simulink model "LKAS"  (R2018b)
settings: Solver=FixedStepDiscrete  StartTime=0.0  StopTime=10.0  FixedStep=0.01  RelTol=1e-3
InitFcn:
  | tmpVer = ver('MATLAB');
  | tmpVer = str2num(tmpVer.Version);
  | % -------------------------------------------------------------------
  | %  MATLAB file generated by Simulink.saveVars on 21-Nov-2019 10:06:14
  | %  MATLAB version: 7.13.0.564 (R2011b)
  | % -------------------------------------------------------------------
  | 
  | 
  | SInt16 = Simulink.AliasType;
  | SInt16.Description = 'Num';
  | if (tmpVer > 7.11)
  | 	SInt16.DataScope = 'Auto';
  | end
  | SInt16.HeaderFile = 'Rte_Type.h';
  | SInt16.BaseType = 'int16';
  | 
  | SInt32 = Simulink.AliasType;
  | SInt32.Description = 'Num';
  | if (tmpVer > 7.11)
  | 	SInt32.DataScope = 'Auto';
  | end
  | SInt32.HeaderFile = 'Rte_Type.h';
  | SInt32.BaseType = 'int32';
  | 
  | SInt8 = Simulink.AliasType;
  | SInt8.Description = 'Num';
  | if (tmpVer > 7.11)
  | 	SInt8.DataScope = 'Auto';
  | end
  | SInt8.HeaderFile = 'Rte_Type.h';
  | SInt8.BaseType = 'int8';
  | 
  | T_A_m2_1024_1_u32 = Simulink.NumericType;
  | T_A_m2_1024_1_u32.Description = 'm2 (square meters  (m2))';
  | if (tmpVer > 7.11)
  | 	T_A_m2_1024_1_u32.DataScope = 'Auto';
  | end
  | T_A_m2_1024_1_u32.HeaderFile = 'Rte_Type.h';
  | T_A_m2_1024_1_u32.DataTypeMode = 'Fixed-point: slope and bias scaling';
  | T_A_m2_1024_1_u32.SignednessBool = false;
  | T_A_m2_1024_1_u32.WordLength = 32;
  | T_A_m2_1024_1_u32.FixedExponent = -10;
  | T_A_m2_1024_1_u32.SlopeAdjustmentFactor = 1;
  | T_A_m2_1024_1_u32.Bias = 0;
  | T_A_m2_1024_1_u32.DataTypeOverride = 'Inherit';
  | T_A_m2_1024_1_u32.IsAlias = true;
  | 
  | T_A_m2_65536_1_u16 = Simulink.NumericType;
  | T_A_m2_65536_1_u16.Description = 'm2 (square meters  (m2))';
  | if (tmpVer > 7.11)
  | 	T_A_m2_65536_1_u16.DataScope = 'Auto';
  | end
  | T_A_m2_65536_1_u16.HeaderFile = 'Rte_Type.h';
  | T_A_m2_65536_1_u16.DataTypeMode = 'Fixed-point: slope and bias scaling';
  | T_A_m2_65536_1_u16.SignednessBool = false;
  | T_A_m2_65536_1_u16.WordLength = 16;
  | T_A_m2_65536_1_u16.FixedExponent = -16;
  | T_A_m2_65536_1_u16.SlopeAdjustmentFactor = 1;
  | T_A_m2_65536_1_u16.Bias = 0;
  | T_A_m2_65536_1_u16.DataTypeOverride = 'Inherit';
  | ... (+4598 lines)
StopFcn:
  | clear  T_A_m2_1024_1_u32 T_A_m2_65536_1_u16 T_A_m2_Float32 T_A_mm2_10_1_u16 T_A_mm2_4_1_s16 T_A_mm2_Float32 T_Cnt_Num_10_1_u32 T_Cnt_Num_1_1_s16 T_Cnt_Num_1_1_s32 T_Cnt_Num_1_1_s8 T_Cnt_Num_1_1_u16 T_Cnt_Num_1_1_u32 T_Cnt_Num_1_1_u8 T_E_J_1_1_s32 T_E_J_Float32 T_E_kJ_128_1_s32 T_E_kJ_Float32 T_E_kwh_10_1_u16 T_E_kwh_Float32 T_Epl_kwhpkm_100_1_u16 T_Epl_kwhpkm_Float32 T_F_N_1_1_s16 T_F_N_Float32 T_I_A_1000_1_u16 T_I_A_1048576_1_s32 T_I_A_2048_1_s16 T_I_A_32_1_s16 T_I_A_Float32 T_I_mA_1_1_s16 T_I_mA_32768_128_s16 T_I_mA_Float32 T_J_kgpm2_128_1_u16 T_J_kgpm2_Float32 T_K_NA_1000_1_s16 T_K_NA_100_1_s16 T_K_NA_100_1_u16 T_K_NA_1024_1_s16 T_K_NA_1024_1_u16 T_K_NA_128_1_s16 T_K_NA_128_1_u16 T_K_NA_128_1_u8 T_K_NA_16777216_1_u32 T_K_NA_16_1_s16 T_K_NA_16_1_u16 T_K_NA_16_1_u8 T_K_NA_1_16_u16 T_K_NA_1_1_s16 T_K_NA_1_1_u16 T_K_NA_1_1_u8 T_K_NA_32768_1_s16 T_K_NA_32768_1_u16 T_K_NA_32_1_s8 T_K_NA_4096_1_u16 T_K_NA_4194304_1_s32 T_K_NA_4194304_1_u16 T_K_NA_65536_1_s32 T_K_NA_65536_1_u16 T_K_NA_8192_1_s16 T_K_NA_8_1_s16 T_K_NA_Float32 T_M_Nm_16_1_s16 T_M_Nm_1_1_s16 T_M_Nm_32768_1_s16 T_M_Nm_32_1_s16 T_M_Nm_4_1_s16 T_M_Nm_512_1_s16 T_M_Nm_Float32 T_P_W_1_4_s16 T_P_W_1_8_s16 T_P_W_Float32 T_P_kW_128_1_s16 T_P_kW_1_8_s16 T_P_kW_8_1_s32 T_P_kW_Float32 T_Pct_pct_1024_1_s32 T_Pct_pct_1024_1_u32 T_Pct_pct_10_1_s16 T_Pct_pct_10_1_u32 T_Pct_pct_128_100_s8 T_Pct_pct_1_1_s16 T_Pct_pct_1_4_u8 T_Pct_pct_255_100_u16 T_Pct_pct_255_100_u8 T_Pct_pct_256_1_s16 T_Pct_pct_256_1_u16 T_Pct_pct_65535_100_u16 T_Pct_pct_Float32 T_R_ohm_1024_1_s16 T_R_ohm_32_1_s16 T_R_ohm_Float32 T_TK_K_16_1_s16 T_TK_K_Float32 T_T_degC_10_400_1_u16 T_T_degC_16_1_s16 T_T_degC_1_40_1_u8 T_T_degC_2_80_1_u8 T_T_degC_Float32 T_U_V_1000_1_u16 T_U_V_10_1_u8 T_U_V_200_1_u8 T_U_V_32_1_s16 T_U_V_4096_1_s16 T_U_V_512_1_s16 T_U_V_65535_8_u16 T_U_V_8192_1_u16 T_U_V_Float32 T_U_mV_1_1_s16 T_U_mV_256_20_u16 T_U_mV_Float32 T_V_l_256_1_s16 T_V_l_4096_1_s16 T_V_l_64_1_s16 T_V_l_65535_100_u16 T_V_l_Float32 T_V_ml_128_1_s16 T_V_ml_1_1_s16 T_V_ml_32768_1_s16 T_V_ml_Float32 T_V_ul_32_1_u16 T_V_ul_Float32 T_Vpl_clpkm_512_1_u16 T_Vpl_clpkm_Float32 T_a_kphps_16_1_s16 T_a_kphps_Float32 T_a_mps2_128_1_s16 T_a_mps2_Float32 T_c_MJpkg_256_1_s16 T_c_MJpkg_Float32 T_c_kJpgpK_1024_1_s16 T_c_kJpgpK_Float32 T_c_kJpkgpK_128_1_u16 T_c_kJpkgpK_Float32 T_chrg_Ah_1_1_s16 T_chrg_Ah_1_1_u16 T_chrg_Ah_1_1_u8 T_chrg_Ah_256_1_u16 T_chrg_Ah_4194304_1_s32 T_chrg_Ah_512_1_u16 T_chrg_Ah_8_1_u16 T_chrg_Ah_Float32 T_cmp_NA_100_1_s16 T_cmp_NA_128_1_s16 T_cmp_NA_16_1_s16 T_cmp_NA_32768_1_u16 T_cmp_NA_Float32 T_d2n_rpmps2_4_1_s16 T_d2n_rpmps2_Float32 T_dPct_pctps_16_1_s16 T_dPct_pctps_256_1_s16 T_dPct_pctps_Float32 T_dT_degCps_128_1_s16 T_dT_degCps_Float32 T_dV_lph_1_1_s16 T_dV_lph_Float32 T_dV_lpm_128_1_s16 T_dV_lpm_32_1_s16 T_dV_lpm_Float32 T_dV_lps_1024_1_u16 T_dV_lps_4_1_u16 T_dV_lps_Float32 T_dV_mlps_1024_1_s16 T_dV_mlps_Float32 T_d_BitField16 T_dm_gps_128_1_s16 T_dm_gps_128_1_u16 T_dm_gps_256_1_u16 T_dm_gps_Float32 T_dm_mgps_1_1_s16 T_dm_mgps_Float32 T_dn_rpmps_1_1_s16 T_dn_rpmps_2_1_s16 T_dn_rpmps_Float32 T_dp_Paps_1_1_s16 T_dp_Paps_Float32 T_dp_kPaps_1_1_s16 T_dp_kPaps_8_1_s16 T_dp_kPaps_Float32 T_dphi_degps_128_1_s16 T_dphi_degps_8_1_s16 T_dphi_degps_Float32 T_dr_ps_256_1_s16 T_dr_ps_Float32 T_drho_mgplps_1_2_s16 T_drho_mgplps_Float32 T_e_NA_1_1_u8 T_f_Hz_1_1_u16 T_f_Hz_1_1_u32 T_f_Hz_64_1_u16 T_f_Hz_8_1_s16 T_f_Hz_Float32 T_g_BitField32 T_l_km_16_1_s16 T_l_km_1_1_u16 T_l_km_1_1_u32 T_l_km_Float32 T_l_m_1024_1_s16 T_l_m_16_1_s16 T_l_m_1_1_u32 T_l_m_Float32 T_l_mm_16_1_s16 T_l_mm_1_1_u16 T_l_mm_4096_1_s16 T_l_mm_4_1_u8 T_l_mm_64_1_s16 T_l_mm_Float32 T_m_g_1_1_s16 T_m_g_2048_1_s16 T_m_g_32_1_u16 T_m_g_Float32 T_m_kg_1024_1_s16 T_m_kg_1_1_s16 T_m_kg_1_1_u32 T_m_kg_Float32 T_m_mg_128_1_s16 T_m_mg_32_1_s16 T_m_mg_Float32 T_n_rpm_1_1_s16 T_n_rpm_1_25_u8 T_n_rpm_256_50_u16 T_n_rpm_2_25_u8 T_n_rpm_4_1_u16 T_n_rpm_Float32 T_p_MPa_64_1_s16 T_p_MPa_Float32 T_p_Pa_1_1_s16 T_p_Pa_Float32 T_p_kPa_1_10_u16 T_p_kPa_1_1_s16 T_p_kPa_1_1_u8 T_p_kPa_256_1_u16 T_p_kPa_32_1_u16 T_p_kPa_64_1_s16 T_p_kPa_Float32 T_phi_deg_100_1_s16 T_phi_deg_1024_1_s16 T_phi_deg_128_1_s16 T_phi_deg_1_1_u8 T_phi_deg_256_1_s16 T_phi_deg_2_1_s8 T_phi_deg_32_1_s16 T_phi_deg_512_6_s32 T_phi_deg_Float32 T_phi_rad_2048_1_s16 T_phi_rad_Float32 T_r_NA_1024_1_s16 T_r_NA_1024_1_u16 T_r_NA_16384_1_s16 T_r_NA_16_1_s16 T_r_NA_256_1_s8 T_r_NA_256_1_u16 T_r_NA_32768_1_u16 T_r_NA_32_1_u16 T_r_NA_4096_1_s16 T_r_NA_65535_2_u16 T_r_NA_8192_1_u16 T_r_NA_Float32 T_rho_gpl_8192_1_s16 T_rho_gpl_Float32 T_rho_kgpm3_16_1_s16 T_rho_kgpm3_Float32 T_rho_mgpl_1_1_s16 T_rho_mgpl_64_1_s16 T_rho_mgpl_Float32 T_t_hour_1_1_s16 T_t_hour_Float32 T_t_m_1_1_u16 T_t_m_Float32 T_t_ms_1_1_s16 T_t_ms_1_1_u16 T_t_ms_1_1_u32 T_t_ms_4096_1_s16 T_t_ms_64_1_s16 T_t_ms_Float32 T_t_s_1000_1_s16 T_t_s_100_1_s16 T_t_s_10_1_s16 T_t_s_10_1_u16 T_t_s_1_1_s16 T_t_s_1_1_u16 T_t_s_1_1_u32 T_t_s_Float32 T_t_us_10_1_u32 T_t_us_1_1_s16 T_t_us_1_1_u32 T_t_us_1_4_u16 T_t_us_Float32 T_v_kph_1_1_u8 T_v_kph_64_1_s16 T_v_kph_64_1_u16 T_v_kph_Float32 T_v_mps_256_1_s16 T_v_mps_Float32 T_w_radps_32_1_s16 T_w_radps_Float32 T_y_BitField8 T_y_BitFieldDiagProgress T_y_BitFieldDiagStatus T_y_NA_1_1_u8 SInt16 SInt32 SInt8 T_BOOLEAN UInt16 UInt32 UInt8 s16 s32 s8 u16 u32 u8
model workspace (MAT data in the model file):
  MCOS : class17 (value not decoded)
  MCOS : class17 (value not decoded)
  MCOS : class17 (value not decoded)
  MCOS : class17 (value not decoded)
  MCOS : class17 (value not decoded)
  MCOS : class17 (value not decoded)
  MCOS : class17 (value not decoded)
  MCOS : class17 (value not decoded)
  MCOS : class17 (value not decoded)
  MCOS : class17 (value not decoded)
  MCOS : class17 (value not decoded)
  MCOS : class17 (value not decoded)
  MCOS : class17 (value not decoded)
  MCOS : class17 (value not decoded)
  MCOS : class17 (value not decoded)
  MCOS : class17 (value not decoded)
  MCOS : class17 (value not decoded)
  MCOS : class17 (value not decoded)
  MCOS : class17 (value not decoded)
  MCOS : class17 (value not decoded)
  MCOS : class17 (value not decoded)
  MCOS : class17 (value not decoded)
  MCOS : class17 (value not decoded)
  MCOS : class17 (value not decoded)
  MCOS : class17 (value not decoded)
  MCOS : class17 (value not decoded)
  MCOS : class17 (value not decoded)
  MCOS : class17 (value not decoded)
  MCOS : class17 (value not decoded)
  MCOS : class17 (value not decoded)
  MCOS : class17 (value not decoded)
  MCOS : class17 (value not decoded)
  MCOS : class17 (value not decoded)
  MCOS : class17 (value not decoded)
  MCOS : class17 (value not decoded)
  MCOS : class17 (value not decoded)
  MCOS : class17 (value not decoded)
  MCOS : class17 (value not decoded)
  MCOS : class17 (value not decoded)
  MCOS : class17 (value not decoded)
  MCOS : class17 (value not decoded)
  MCOS : class17 (value not decoded)
  MCOS : class17 (value not decoded)
  MCOS : class17 (value not decoded)
  MCOS : class17 (value not decoded)
  MCOS : class17 (value not decoded)
  MCOS : class17 (value not decoded)
  MCOS : class17 (value not decoded)
  MCOS : class17 (value not decoded)
  MCOS : class17 (value not decoded)
  MCOS : class17 (value not decoded)
  MCOS : class17 (value not decoded)
  MCOS : class17 (value not decoded)
  MCOS : class17 (value not decoded)
  MCOS : class17 (value not decoded)
  MCOS : class17 (value not decoded)
  MCOS : class17 (value not decoded)
  MCOS : class17 (value not decoded)
  MCOS : class17 (value not decoded)
  MCOS : class17 (value not decoded)
  MCOS : class17 (value not decoded)
  MCOS : class17 (value not decoded)
  MCOS : class17 (value not decoded)
  MCOS : class17 (value not decoded)
  MCOS : class17 (value not decoded)
  MCOS : class17 (value not decoded)
  MCOS : class17 (value not decoded)
  MCOS : class17 (value not decoded)
  MCOS : class17 (value not decoded)
  MCOS : class17 (value not decoded)
  MCOS : class17 (value not decoded)
  MCOS : class17 (value not decoded)
  MCOS : class17 (value not decoded)
  MCOS : class17 (value not decoded)
  MCOS : class17 (value not decoded)
  MCOS : class17 (value not decoded)
  MCOS : class17 (value not decoded)
  MCOS : class17 (value not decoded)
  MCOS : class17 (value not decoded)
  MCOS : class17 (value not decoded)
  MCOS : class17 (value not decoded)
  MCOS : class17 (value not decoded)
  MCOS : class17 (value not decoded)
  MCOS : class17 (value not decoded)
  MCOS : class17 (value not decoded)
  MCOS : class17 (value not decoded)
  MCOS : class17 (value not decoded)
  MCOS : class17 (value not decoded)
  MCOS : class17 (value not decoded)
undefined symbols (not defined in the file): LKA_CarWidth, LKA_SampleTime, LKA_StrRatio_C, LKA_Veh2CamL_C, LKA_Veh2CamW_C, LKA_WhlBaseL_C, LL_CompSWA_C, LL_CrvtPrvwT_C, LL_DesDvt_C, LL_DvtComp_C, LL_DvtPrvwT_C, LL_DvtSpdDet_vDvtSpdMin_C, LL_HdAgExT_C, LL_HdAgPrvwT_C, LL_LAccMax_C, LL_LAccRMax_C, LL_LDW_EarliestWarnLine_C, LL_LDW_LatestWarnLine_C, LL_LDWS_SUPPRESS_HEADING, LL_LFClb_TFC_DiffCtlBalance, LL_LFClb_TFC_DiffCtrlMaxSWA, LL_LFClb_TFC_DiffCtrlRatio, LL_LFClb_TFC_facmGainLutGain1_C, LL_LFClb_TFC_facmGainLutGain2_C, LL_LFClb_TFC_facmIntegRatio, LL_LFClb_TFC_facmKlat_C, LL_LFClb_TFC_FfCtlRatio_C, LL_LFClb_TFC_phiIntegCtlMaxSWA_C, LL_LFClb_TFC_tiKlatPrvwT_C, LL_LFClb_TFC_vGainLutVehSpdLwr_C, LL_LFClb_TFC_vGainLutVehSpdUpr_C, LL_LKA_EarliestWarnLine_C, LL_LKA_LatestWarnLine_C, LL_LKAExPrcs_ExitC0Dvt, LL_LKAExPrcs_ExitC0Swt, LL_LKAExPrcs_tiExitTime1, LL_LKAExPrcs_tiExitTime2, LL_LKAExPrcs_tiExitTime3, LL_LKAS_OUT_OF_CONTROL_LAT_VEL, LL_LKAS_OUT_OF_CONTROL_TTLC, LL_LKASWASyn_M0, LL_LKASWASyn_M1, LL_LKASWASyn_M2, LL_LKASWASyn_M3K, LL_LKASWASyn_SWAaddMax, LL_LKASWASyn_T2, LL_LKASWASyn_tiTrqSwaRtTime, LL_LKASWASyn_tiTrqSwaTime, LL_LKASWASyn_TrqMax, LL_LKASWASyn_TrqSwaAddSwt, LL_LKASWASyn_TrqSwaRateDiff, LL_LSpdCompT_C, LL_lStpLngth_C, LL_MAX_DELAY_EPSSTAR_TIME, LL_MAX_DRIVER_TORQUE_DISABLE, LL_MAX_DRIVER_TORQUE_ENABLE, LL_MAX_LANE_WIDTH_DISABLE, LL_MAX_LANE_WIDTH_ENABLE, LL_MAX_LAT_ACC_DISABLE, LL_MAX_LAT_ACC_ENABLE ... (+29)
libraries: simulink x190, dspstat3 x3, simulink_extras x1
(part 7 of 19)

== system LKAS/LKAS/LL/LL Inputs Mapping/bsLaneInfo/LanesReconstruct  ==
  bsL0Info : Inport
  bsR0Info : Inport  Port=2
  bsL1Info : Inport  Port=3
  bsR1Info : Inport  Port=4
  Bus Selector5 : BusSelector  OutputSignals=L0_Q
  Bus Selector6 : BusSelector  OutputSignals=R0_Q
  LaneReconstructSM : Stateflow chart  TreatAsAtomicUnit=on
  Left 1Lane Reconstruct (Lft1LaneR) : Subsystem
  Left Lane Reconstruct (LftLaneR) : Subsystem
  Right 1Lane Reconstruct (Rgt1LaneR) : Subsystem
  Right Lane Reconstruct (RgtLaneR) : Subsystem
  RoadSide Offset : Subsystem
  Switch : Switch  Criteria=u2 > Threshold
  Switch1 : Switch  Criteria=u2 > Threshold
  bsL0InfoR : Outport
  bsR0InfoR : Outport  Port=2
  bsL1InfoR : Outport  Port=3
  bsR1InfoR : Outport  Port=4
  wires:
  RoadSide Offset/2(bsR0Infoout) -> Bus Selector6/1, Left Lane Reconstruct (LftLaneR)/2(bsR0Info), Right Lane Reconstruct (RgtLaneR)/2(bsR0Info), Switch/1
  RoadSide Offset/1(bsL0Infoout) -> Bus Selector5/1, Right Lane Reconstruct (RgtLaneR)/1(bsL0Info), Switch1/1, Left Lane Reconstruct (LftLaneR)/3(bsL0Info)
  bsL0Info/1 -> RoadSide Offset/1(bsL0Info)
  bsR0Info/1 -> RoadSide Offset/2(bsR0Info)
  [LftFlg] -> Switch1/2
  [RgtFlg] -> Switch/2
  [LftFlg] -> Left 1Lane Reconstruct (Lft1LaneR)/1(stFlag)
  [RgtFlg] -> Right 1Lane Reconstruct (Rgt1LaneR)/1(stFlag)
  Left 1Lane Reconstruct (Lft1LaneR)/1(bsL1InfoR) -> bsL1InfoR/1
  Right 1Lane Reconstruct (Rgt1LaneR)/1(bsL1InfoR) -> bsR1InfoR/1
  bsR1Info/1 -> Right 1Lane Reconstruct (Rgt1LaneR)/2(bsR1Info)
  LaneReconstructSM/3(LaneRSM_stRgtFlg) -> [RgtFlg]
  LaneReconstructSM/2(LaneRSM_stLftFlg) -> [LftFlg]
  LaneReconstructSM/1(LaneRSM_stRoadFlg) -> [RoadFlg]
  Switch1/1 -> bsL0InfoR/1
  Switch/1 -> bsR0InfoR/1
  Right Lane Reconstruct (RgtLaneR)/1(bsR0InfoR) -> Switch/3
  Left Lane Reconstruct (LftLaneR)/1(bsL0InfoR) -> Switch1/3
  RoadSide Offset/3(lRoadW) -> Right Lane Reconstruct (RgtLaneR)/3(lRoadW), Left Lane Reconstruct (LftLaneR)/1(lRoadW), [RoadWidth]
  Bus Selector5/1 -> LaneReconstructSM/1(LaneRSM_stL0Ql)  "<L0_Q>"
  Bus Selector6/1 -> LaneReconstructSM/2(LaneRSM_stR0Ql)  "<R0_Q>"
  bsL1Info/1 -> Left 1Lane Reconstruct (Lft1LaneR)/2(bsL1Info)

== system LKAS/LKAS/LL/LLOn/LDW/Heading Angle Detection (HdAgDet) ==
  HdAgDet_stLDWActvFlg : Inport
  HdAgDet_phiHdAgLft : Inport  Port=2
  HdAgDet_phiHdAgRgt : Inport  Port=3
  HdAgDet_phiHdAgThres_C : Inport  Port=4
  Constant : Constant  Value=5  OutDataTypeStr=single
  If : If  IfExpression=u1==1  ElseIfExpressions=u1==2
  If Action Subsystem : Subsystem  TreatAsAtomicUnit=on
  If Action Subsystem1 : Subsystem  TreatAsAtomicUnit=on
  If Action Subsystem2 : Subsystem  TreatAsAtomicUnit=on
  Merge : Merge  Inputs=3  InitialOutput=0
  Relational Operator : RelationalOperator  OutDataTypeStr=boolean  RndMeth=Nearest
  Sum Condition : Subsystem
  HdAgDet_stHdAgDetFlg : Outport
  wires:
  If/1 -> If Action Subsystem/Action
  If Action Subsystem/1(Out1) -> Merge/1
  If Action Subsystem1/1(Out1) -> Merge/2
  If/2 -> If Action Subsystem1/Action
  If Action Subsystem2/1(Out1) -> Merge/3
  If/3 -> If Action Subsystem2/Action
  HdAgDet_phiHdAgLft/1 -> If Action Subsystem/1(In1)
  HdAgDet_phiHdAgRgt/1 -> If Action Subsystem1/1(In1)
  HdAgDet_stLDWActvFlg/1 -> If/1
  Merge/1 -> Relational Operator/1
  HdAgDet_phiHdAgThres_C/1 -> Relational Operator/2
  Sum Condition/1(Out) -> HdAgDet_stHdAgDetFlg/1
  Relational Operator/1 -> Sum Condition/1(In), Sum Condition/Enable
  Constant/1 -> Sum Condition/2(Sum)

== system LKAS/LKAS/LL/LLOn/LKA/Driver Torque Addition (DTA) ==
  DTA_bsInInfoSyn : Inport
  DTA_bsLFClb : Inport  Port=2
  Bus Selector : BusSelector  OutputSignals=LL_LKASWAClb.LL_LKASWASyn_TrqSwaAddSwt
  Compare To Constant : simulink/Logic and Bit Operations/Compare To Constant  relop=>  const=0  OutDataTypeStr=boolean
  Subsystem : Subsystem
  Subsystem1 : Subsystem
  DTA_phiDTASWACmd : Outport
  DTA_M : Outport  Port=2
  wires:
  [LKA_SampleTime] -> Subsystem/3(LKA_SampleTime)
  DTA_bsInInfoSyn/1 -> Subsystem/1(DTA_bsInInfoSyn), Subsystem1/1(DTA_bsInInfoSyn)
  DTA_bsLFClb/1 -> Subsystem1/2(DTA_bsLFClb), Subsystem/2(DTA_bsLFClb), Bus Selector/1
  Subsystem/1(Out1) -> DTA_phiDTASWACmd/1
  Subsystem1/1(Out1) -> DTA_M/1
  Bus Selector/1 -> Compare To Constant/1  "<LL_LKASWASyn_TrqSwaAddSwt>"
  Compare To Constant/1 -> Subsystem/Enable

== system LKAS/LKAS/LL/LLOn/LKA/LKA Exit Processing (LKAExPrcs) ==
  LKAExPrcs_bsInInfoSyn : Inport
  LKAExPrcs_bsLKAInPInfo : Inport  Port=2
  LKAExPrcs_bsLKAClb : Inport  Port=3
  LKAExPrcs_PlanT1 : Inport  Port=4
  Cast To Single : DataTypeConversion  OutDataTypeStr=single
  Exit Time 1 : Subsystem
  Exit Time 2 : Subsystem
  Exit Time 3 : Subsystem
  Fcn : Fcn  Expr=u(3)*(u(3)==1)*3+u(2)*(u(3)==0)*2+u(1)*(u(2)==0&&u(3)==0)
  Logical Operator3 : Logic  Operator=OR  Inputs=3  AllPortsSameDT=off  OutDataTypeStr=boolean
  Mux : Mux  Inputs=3
  LKAExPrcs_stExFlg : Outport
  LKAExPrcs_stExNum : Outport  Port=2
  wires:
  LKAExPrcs_bsInInfoSyn/1 -> Exit Time 3/1(bsInInfoSyn), Exit Time 2/1(bsInInfoSyn)
  Logical Operator3/1 -> LKAExPrcs_stExFlg/1
  Exit Time 1/1(Exit1) -> Mux/1, Logical Operator3/1
  Exit Time 2/1(Exit2) -> Mux/2, Logical Operator3/2
  Exit Time 3/1(Exit3) -> Mux/3, Logical Operator3/3
  LKAExPrcs_bsLKAInPInfo/1 -> Exit Time 3/2(bsLKAInPInfo), Exit Time 2/3(bsLKAInPInfo), Exit Time 1/1(bsLKAInPInfo)
  LKAExPrcs_bsLKAClb/1 -> Exit Time 1/2(bsLKAClb), Exit Time 2/2(bsLKAClb), Exit Time 3/3(bsLKAClb)
  LKAExPrcs_PlanT1/1 -> Exit Time 2/4(T1), Exit Time 3/4(T1)
  Mux/1 -> Cast To Single/1
  Fcn/1 -> LKAExPrcs_stExNum/1  "ExNum"
  Cast To Single/1 -> Fcn/1

== system LKAS/LKAS/LL/LLOn/LKA/LKA Motion Planning (LKAMP)  ==
  LKAMP_bsInInfoSyn : Inport
  LKAMP_stLKAActvFlg : Inport  Port=2
  LKAMP_bsLKAInPInfo : Inport  Port=3
  LKAMP_bsLKAClb : Inport  Port=4
  LLClb_bsConstantClb : Inport  Port=5
  Add : Sum  OutDataTypeStr=uint8
  Bus Selector : BusSelector  OutputSignals=MPInP_vVehSpdIni
  Bus Selector1 : BusSelector  OutputSignals=bsVehMovInfo.ESC_VehSpd
  Bus Selector2 : BusSelector  OutputSignals=LKA_CarWidth
  Bus Selector3 : BusSelector  OutputSignals=LL_HdAgExT_C,LL_LSpdCompT_C
  Bus Selector4 : BusSelector  OutputSignals=bsVehMovInfo.ESC_VehSpd
  Bus Selector5 : BusSelector  OutputSignals=LW_LaneWidth
  Constant : Constant  OutDataTypeStr=uint8  SampleTime=-1
  Constant19 : Constant  OutDataTypeStr=uint8  SampleTime=-1
  If : If  NumInputs=2  IfExpression=u1==u2  ShowElse=off
  LKA Motion Planning Calculation (LKAMPCal) : Subsystem  Description=|
      | Block Name: LKA Motion Planning Calculation
      | Ab.: LKAMPCal
      | No.: 1.2.3.2
      | Rev: 0.0.1
      | Update Date: 19-3-26
      settings: RTWSystemCode=Nonreusable function
  Memory1 : Memory  InheritSampleTime=on
  Motion Planning Input Processing (MPInP) : Subsystem  Description=|
      | Block Name: Motion Planning Input Processing
      | Ab.: MPInP
      | No.: 1.2.3.1
      | Rev: 0.0.1
      | Update Date: 19-3-26
  Nominal Time Calculation (NomTCalc) : Subsystem  Description=|
      | Block Name: Nominal Time Calculation
      | Ab.: NomTCalc
      | No.: 1.2.3.3
      | Rev: 0.0.1
      | Update Date: 19-3-26
  Saturation1 : Saturate  UpperLimit=5  LowerLimit=0  OutDataTypeStr=uint8
  Saturation6 : Saturate  UpperLimit=2  LowerLimit=0.2
  Steering Wheel Angle Command Calculation (SWACmdCal) : Subsystem  Description=|
      | Block Name: Steering Wheel Angle Command Calculation
      | Ab.: SWACmdCal
      | No.: 1.2.3.4
      | Rev: 0.0.1
      | Update Date: 19-3-26
  Switching Condition (SwtCon) : Subsystem
  LKAMP_phiSWACmd : Outport
  LKAMP_tiT1 : Outport  Port=2
  LKAMP_tiT2 : Outport  Port=3
  wires:
  Steering Wheel Angle Command Calculation (SWACmdCal)/3(SWACmdCal_tiT2) -> LKAMP_tiT2/1
  Motion Planning Input Processing (MPInP)/1(MPInP_bsMPInPInfo) -> Steering Wheel Angle Command Calculation (SWACmdCal)/2(SWACmdCal_bsLKAInPInfo), Bus Selector/1, LKA Motion Planning Calculation (LKAMPCal)/1(LKAMPCal_bsLKAInPInfo)  "LKAMP_bsMPInPInfo"
  Steering Wheel Angle Command Calculation (SWACmdCal)/2(SWACmdCal_tiT1) -> Saturation6/1
  Steering Wheel Angle Command Calculation (SWACmdCal)/1(SWACmdCal_phiSWACmd) -> LKAMP_phiSWACmd/1
  Bus Selector/1 -> Nominal Time Calculation (NomTCalc)/2(NomTCalc_vVehSpdIni)  "<MPInP_vVehSpdIni>"
  Bus Selector1/1 -> Nominal Time Calculation (NomTCalc)/1(NomTCalc_vVehSpd)  "<ESC_VehSpd>"
  Nominal Time Calculation (NomTCalc)/1(NomTCalc_tiNomT) -> Steering Wheel Angle Command Calculation (SWACmdCal)/3(SWACmdCal_tiNomT)
  Switching Condition (SwtCon)/1(SwtCon_phiHdAgMax) -> Motion Planning Input Processing (MPInP)/2(MPInP_phiHdAgMax)
  LKA Motion Planning Calculation (LKAMPCal)/1(LKAMPCal_bsLKAMPCalOut) -> Steering Wheel Angle Command Calculation (SWACmdCal)/1(SWACmdCal_bsK1K2DetOut)
  If/1 -> LKA Motion Planning Calculation (LKAMPCal)/Action
  Memory1/1 -> Add/2
  Constant/1 -> Add/1
  Constant19/1 -> If/2
  Add/1 -> Saturation1/1
  Saturation1/1 -> Memory1/1, If/1
  Bus Selector3/1 -> Switching Condition (SwtCon)/6(SwtCon_tiHdAgExTime_C)  "<LL_HdAgExT_C>"
  Bus Selector4/1 -> Switching Condition (SwtCon)/3(SwtCon_vVehSpd)  "<ESC_VehSpd>"
  LKAMP_stLKAActvFlg/1 -> Switching Condition (SwtCon)/1(SwtCon_stLKAActvFlg), Motion Planning Input Processing (MPInP)/1(MPInP_stLKAActvFlg)
  LKAMP_bsLKAClb/1 -> Bus Selector3/1, LKA Motion Planning Calculation (LKAMPCal)/2(LKAMPCal_bsLKAClb)
  Bus Selector2/1 -> Switching Condition (SwtCon)/5(SwtCon_lCarWidth_C)  "<LKA_CarWidth>"
  LKAMP_bsLKAInPInfo/1 -> Bus Selector5/1, Switching Condition (SwtCon)/2(SwtCon_bsLKAInPInfo), Motion Planning Input Processing (MPInP)/3(MPInP_bsLKAInPInfo)
  LLClb_bsConstantClb/1 -> LKA Motion Planning Calculation (LKAMPCal)/3(LLClb_bsConstantClb), Bus Selector2/1
  Bus Selector3/2 -> Switching Condition (SwtCon)/7(SwtCon_tiLSpdCompT_C)  "<LL_LSpdCompT_C>"
  LKAMP_bsInInfoSyn/1 -> Motion Planning Input Processing (MPInP)/4(MPInP_bsInInfoSyn), Bus Selector1/1, Bus Selector4/1
  Saturation6/1 -> LKAMP_tiT1/1
  Bus Selector5/1 -> Switching Condition (SwtCon)/4(SwtCon_lLaneWidth_C)  "<LW_LaneWidth>"

== system LKAS/LKAS/LL/LLOn/LKA/LKA SWA Limit (LKASWALim) ==
  LKASWALim_phiTFCSWACmd : Inport
  LKASWALim_Ff : Inport  Port=2
  LKASWALim_bsLKAInPInfo : Inport  Port=3
  LKASWALim_bsLKAClb : Inport  Port=4
  Add : Sum  Inputs=+-+  OutDataTypeStr=single
  Add1 : Sum
  Add2 : Sum
  Bus Selector1 : BusSelector  OutputSignals=LKAInP_phiSWAPos,UndrLim_phiSWAMax,UndrLim_dphiSWARMax
  Bus Selector3 : BusSelector  OutputSignals=LL_CompSWA_C
  Gain1 : Gain  Gain=-1.4  OutDataTypeStr=single
  Gain2 : Gain  Gain=-1  OutDataTypeStr=single
  Gain3 : Gain  Gain=1.4  OutDataTypeStr=single
  "Rate Limiter Dynamic " : Subsystem
  Saturation Dynamic : simulink/Discontinuities/Saturation Dynamic  OutMin=[]  OutMax=[]  OutDataTypeStr=Inherit: Same as second input  OutDataType=fixdt(1, 16)  OutScaling=2^-10  DoSatur=off
  LKASWALim_phiSWACmd : Outport
  wires:
  Gain3/1 -> "Rate Limiter Dynamic "/1(up)
  Saturation Dynamic/1 -> "Rate Limiter Dynamic "/2(u)
  "Rate Limiter Dynamic "/1(Y) -> LKASWALim_phiSWACmd/1
  Bus Selector3/1 -> Add/2  "<LL_CompSWA_C>"
  LKASWALim_phiTFCSWACmd/1 -> Add/1
  LKASWALim_bsLKAClb/1 -> Bus Selector3/1
  Bus Selector1/2 -> Add1/2, Gain2/1  "<UndrLim_phiSWAMax>"
  Bus Selector1/3 -> Gain3/1, Gain1/1  "<UndrLim_dphiSWARMax>"
  Gain2/1 -> Add2/2
  Gain1/1 -> "Rate Limiter Dynamic "/3(lo)
  Add/1 -> Saturation Dynamic/2
  LKASWALim_bsLKAInPInfo/1 -> Bus Selector1/1
  Bus Selector1/1 -> Add/3  "<LKAInP_phiSWAPos>"
  LKASWALim_Ff/1 -> Add2/1, Add1/1
  Add1/1 -> Saturation Dynamic/1
  Add2/1 -> Saturation Dynamic/3

== system LKAS/LKAS/LL/LLOn/LKA/Lane Following (LF) ==
  LF_bsInInfoSyn : Inport
  LF_bsLKAInPInfo : Inport  Port=2
  LF_bsLFClb : Inport  Port=3
  LF_bsConstantClb : Inport  Port=4
  Bus Selector4 : BusSelector  OutputSignals=LL_TFCClb
  Preview Information Calculation (PIC) : Subsystem  Description=|
      | Block Name:Preview Information Calculation
      | Ab.: PIC
      | No.: 02.01
      | Rev: 00.00.01
      | Update Date: 19-3-28
  Trajectory Following Control (TFC) : Subsystem  Description=|
      | Block Name:Trajectory Following Control
      | Ab.: TFC
      | No.: 02.02
      | Rev: 00.00.01
      | Update Date: 19-3-28
  LF_phiFfLFSWACmd : Outport
  LF_phiPropSWACmd : Outport  Port=2
  LF_phiIntegSWACmd : Outport  Port=3
  LF_phiDiffSWACmd : Outport  Port=4
  wires:
  Trajectory Following Control (TFC)/4(TFC_phiDiffSWACmd) -> LF_phiDiffSWACmd/1
  Trajectory Following Control (TFC)/3(TFC_phiIntegSWACmd) -> LF_phiIntegSWACmd/1
  Trajectory Following Control (TFC)/2(TFC_phiPropSWACmd) -> LF_phiPropSWACmd/1
  LF_bsConstantClb/1 -> Trajectory Following Control (TFC)/4(TFC_bsConstantClb)
  LF_bsLFClb/1 -> Bus Selector4/1
  Bus Selector4/1 -> Trajectory Following Control (TFC)/3(TFC_bsTFCClb)  "<LL_TFCClb>"
  Preview Information Calculation (PIC)/1(PIC_bsPrvwInfo) -> Trajectory Following Control (TFC)/1(TFC_bsPrvwInfo)
  LF_bsInInfoSyn/1 -> Trajectory Following Control (TFC)/2(TFC_bsInInfoSyn)
  Trajectory Following Control (TFC)/1(TFC_phiFfSWACmd) -> LF_phiFfLFSWACmd/1
  LF_bsLKAInPInfo/1 -> Preview Information Calculation (PIC)/1(PIC_bsLKAInPInfo)

== system LKAS/LKAS/LL/LLOn/LKA/Plan To LaneFollowing (PTLF) ==
  InP : Inport
  Plan : Inport  Port=2
  T1 : Inport  Port=3
  DrvTrq : Inport  Port=4
  Ff : Inport  Port=5
  P : Inport  Port=6
  I : Inport  Port=7
  D : Inport  Port=8
  Add1 : Sum  Inputs=+-
  Add2 : Sum  Inputs=+-
  Add3 : Sum
  Add4 : Sum  Inputs=+++++
  Add5 : Sum  Inputs=+-
  Bus Selector1 : BusSelector  OutputSignals=Pr_bsPrInfo.bsPrCrvtInfo.crPrvwCrvt
  Bus Selector2 : BusSelector  OutputSignals=Pr_bsPrInfo.bsPrHdAgInfo.phiHdAgLft,Pr_bsPrInfo.bsPrHdAgInfo.phiHdAgRgt
  Constant1 : Constant  Value=0.1  OutDataTypeStr=single
  Constant2 : Constant  OutDataTypeStr=single
  Divide : Product  Inputs=*/
  Divide{1..2,5..7} (5 alike) : Product  Inputs=**
  Divide3 : Product  Inputs=*/
  Divide4 : Product  Inputs=*/
  InsideJudge : Subsystem
  InsideJudge1 : Subsystem
  LowPass : Subsystem
  Saturation : Saturate  UpperLimit=1  LowerLimit=0
  Saturation1 : Saturate  UpperLimit=1  LowerLimit=0
  Saturation2 : Saturate  UpperLimit=1  LowerLimit=0
  Saturation3 : Saturate  UpperLimit=0.004  LowerLimit=-0.004
  Saturation6 : Saturate  LowerLimit=0.2
  Switch : Switch  Criteria=u2 > Threshold
  TickTime (TTime) : Subsystem
      mask Display:
      | port_label('output', 1, 'TTime');
      | color('blue');
      | text(0.98,0.9,'VCDC Block','horizontalAlignment','right');
      | color('black');
      | text(0.5,0.55,'Tick Time','horizontalAlignment','center');
      | text(0.5,0.4,'(TTime)','horizontalAlignment','center');
  TimeGain : Subsystem
  SWACmd : Outport
  wires:
  Constant1/1 -> LowPass/1(T)
  [LKA_SampleTime] -> LowPass/3(dT)
  LowPass/1(y) -> SWACmd/1
  Divide2/1 -> Add4/3  "S_D"
  Divide4/1 -> Saturation1/1
  Divide1/1 -> Add4/2  "S_PI"
  Add3/1 -> Divide1/2
  I/1 -> Add3/2
  P/1 -> Add3/1
  Divide7/1 -> Add4/1  "S_Plan"
  DrvTrq/1 -> Divide6/1
  D/1 -> Divide2/1
  Ff/1 -> Divide5/2
  Add5/1 -> Divide7/2
  Divide6/1 -> Add4/5  "S_DT"
  [Plan] -> Divide7/1
  Saturation2/1 -> Divide1/1, Add5/2
  Constant2/1 -> Add5/1
  Saturation/1 -> Divide6/2
  Divide/1 -> Saturation2/1
  Divide3/1 -> Saturation/1
  [T1] -> Add2/2
  Add2/1 -> Divide/1
  Add4/1 -> LowPass/2(u)
  [TFC] -> Divide/2
  Saturation1/1 -> Divide2/2
  Bus Selector1/1 -> Saturation3/1  "<crPrvwCrvt>"
  Saturation3/1 -> InsideJudge/2(Crvt)
  Divide5/1 -> Switch/3, Switch/1
  TimeGain/1(Out1) -> Divide5/1
  TickTime (TTime)/1(Out1) -> [Time]
  [ActFlg] -> InsideJudge/1(Flg)
  InsideJudge/1(Out1) -> Switch/2
  Switch/1 -> Add4/4  "S_Ff"
  [Time] -> Divide3/1
  [Time] -> Add2/1
  [T1] -> Divide3/2
  InsideJudge1/1(T1_1) -> [T1], Saturation6/1
  Saturation6/1 -> [TFC]
  [Time] -> TimeGain/1(Time)
  [T1] -> TimeGain/2(T1)
  [TFC] -> TimeGain/3(TFC)
  [T1] -> Add1/2
  [TFC] -> Divide4/2
  Add1/1 -> Divide4/1
  [Time] -> Add1/1
  InP/1 -> Bus Selector2/1, Bus Selector1/1
  [ActFlg] -> InsideJudge1/1(Flg)
  Bus Selector2/1 -> InsideJudge1/2(HdAgLft)  "<phiHdAgLft>"
  Bus Selector2/2 -> InsideJudge1/3(HdAgRgt)  "<phiHdAgRgt>"
  T1/1 -> InsideJudge1/4(T1)
  Plan/1 -> InsideJudge1/5(Plan)
  [Time] -> InsideJudge1/6(Time)
  InsideJudge1/2(Plan_1) -> [Plan]

== system LKAS/LKAS/LL/LLOn/LKA Input Processing (LKAInP)/Lane Width Calculation (LW) ==
  LW_bsInInfoSyn : Inport
  Abs : Abs
  Abs1 : Abs
  Add : Sum
  Bus Selector : BusSelector  OutputSignals=bsLaneInfo.bsL0Info.L0_C0,bsLaneInfo.bsR0Info.R0_C0
  Saturation : Saturate  UpperLimit=6  LowerLimit=2
  LW_LaneWidth : Outport
  wires:
  LW_bsInInfoSyn/1 -> Bus Selector/1
  Bus Selector/1 -> Abs/1  "<L0_C0>"
  Bus Selector/2 -> Abs1/1  "<R0_C0>"
  Abs/1 -> Add/1
  Abs1/1 -> Add/2
  Add/1 -> Saturation/1
  Saturation/1 -> LW_LaneWidth/1  "LaneWidth"

== system LKAS/LKAS/LL/LLOn/LKA Input Processing (LKAInP)/Predicted Deviation Calculation (PrDvt) ==
  PrdcDvt_stLKAActvFlg : Inport
  PrdcDvt_bsInInfoSyn : Inport  Port=2
  PrdcDvt_bsPrdcHdAgInfo : Inport  Port=3
  PrdcDvt_bsLKAClb : Inport  Port=4
  Bus Creator1 : BusCreator  Inputs=8
  Bus Selector : BusSelector  OutputSignals=bsLaneInfo.bsL0Info,bsVehMovInfo.ESC_VehSpd,bsLaneInfo.bsR0Info
  Bus Selector1 : BusSelector  OutputSignals=LL_DvtPrvwT_C,LL_DvtComp_C
  Bus Selector2 : BusSelector  OutputSignals=bsLaneInfo.bsL0Info.L0_C0,bsLaneInfo.bsR0Info.R0_C0
  Bus Selector3 : BusSelector  OutputSignals=EnaCClb.LL_DvtComp_C
  Lane Information Selection (LaneInfoSel) : Subsystem
  Lane Information Selection (LaneInfoSel)1 : Subsystem
  Left Front Conner Deviation Calculation (LFCDvtCalc) : Subsystem
  Predicted Deviation Correction (PrdcDvtCor) : Subsystem
  Predicted Deviation of Left Lane Line (PrdcDvtLft) : Subsystem
  Predicted Deviation of Left Line (PrdcDvtLft) : Subsystem
  Predicted Deviation of Right  Line (PrdcDvtRgt) : Subsystem
  Predicted Deviation of Right Lane Line (PrdcDvtRgt) : Subsystem
  Right Front Conner Deviation Calculation (RFCDvtCalc) : Subsystem
  Z Calculation (ZCalc) : Subsystem
  PrdcDvt_bsPrdcDvtInfo : Outport
  wires:
  Bus Selector1/2 -> Predicted Deviation of Left Line (PrdcDvtLft)/4(PrdcDvtLft_lDvtComp_C), Predicted Deviation of Right  Line (PrdcDvtRgt)/4(PrdcDvtLft_lDvtComp_C)  "<LL_DvtComp_C>"
  Bus Selector1/1 -> Z Calculation (ZCalc)/2(ZCalc_tiDvtPrvwT_C)  "<LL_DvtPrvwT_C>"
  PrdcDvt_bsLKAClb/1 -> Bus Selector1/1
  Predicted Deviation Correction (PrdcDvtCor)/1(PrdcDvtCor_lPrdcDvtCor) -> Predicted Deviation of Right  Line (PrdcDvtRgt)/2(PrdcDvtLft_lPrdcDvtCor), Predicted Deviation of Left Line (PrdcDvtLft)/2(PrdcDvtLft_lPrdcDvtCor)
  PrdcDvt_bsPrdcHdAgInfo/1 -> Right Front Conner Deviation Calculation (RFCDvtCalc)/3(PrdcDvt_bsPrHdAgInfo), Left Front Conner Deviation Calculation (LFCDvtCalc)/1(PrdcDvt_bsPrHdAgInfo), Predicted Deviation Correction (PrdcDvtCor)/1(PrdcDvtCor_bsPrdcHdAgInfo), Predicted Deviation of Right  Line (PrdcDvtRgt)/1(PrdcDvtLft_bsPrdcHdAgInfo), Predicted Deviation of Left Line (PrdcDvtLft)/1(PrdcDvtLft_bsPrdcHdAgInfo)
  Bus Selector/1 -> Predicted Deviation of Left Lane Line (PrdcDvtLft)/1(PrdcDvtLft_bsL0Info)  "<bsL0Info>"
  PrdcDvt_bsInInfoSyn/1 -> Bus Selector2/1, Bus Selector/1
  Z Calculation (ZCalc)/1(ZCalc_lPrvwDstZ) -> Predicted Deviation of Right Lane Line (PrdcDvtRgt)/1(PrdcDvtRgt_lPrvwDstZ), Predicted Deviation of Left Lane Line (PrdcDvtLft)/2(PrdcDvtLft_lPrvwDstZ), Predicted Deviation Correction (PrdcDvtCor)/2(PrdcDvtCor_lPrvwDstZ)
  Predicted Deviation of Right Lane Line (PrdcDvtRgt)/1(PrdcDvtRgt_lPrdcDvtRgt) -> Bus Creator1/5, Predicted Deviation of Right  Line (PrdcDvtRgt)/3(PrdcDvtLft_lPrdcDvtLft)  "lPrvwDvtRgt"
  Bus Selector/2 -> Z Calculation (ZCalc)/1(ZCalc_vVehSpd)  "<ESC_VehSpd>"
  Bus Selector/3 -> Predicted Deviation of Right Lane Line (PrdcDvtRgt)/2(PrdcDvtRgt_bsR0Info)  "<bsR0Info>"
  Predicted Deviation of Left Lane Line (PrdcDvtLft)/1(PrdcDvtLft_lPrdcDvtLft) -> Bus Creator1/4, Predicted Deviation of Left Line (PrdcDvtLft)/3(PrdcDvtLft_lPrdcDvtLft)  "lPrvwDvtLft"
  Predicted Deviation of Left Line (PrdcDvtLft)/1(PrdcDvtLft_lDvtLft) -> Bus Creator1/2, Lane Information Selection (LaneInfoSel)/2(LaneInfoSel_facmLftLane)  "lPrdcDvtLft"
  Predicted Deviation of Right  Line (PrdcDvtRgt)/1(PrdcDvtLft_lDvtRgt) -> Lane Information Selection (LaneInfoSel)/3(LaneInfoSel_facmRgtLane), Bus Creator1/3  "lPrdcDvtRgt"
  Bus Creator1/1 -> PrdcDvt_bsPrdcDvtInfo/1
  PrdcDvt_stLKAActvFlg/1 -> Lane Information Selection (LaneInfoSel)/1(LaneInfoSel_stLKAActvFlg), Lane Information Selection (LaneInfoSel)1/1(LaneInfoSel_stLKAActvFlg)
  Lane Information Selection (LaneInfoSel)/1(LaneInfoSel_facmActvLane) -> Bus Creator1/1  "lPrdcDvt"
  Bus Selector2/1 -> Left Front Conner Deviation Calculation (LFCDvtCalc)/2(LFCDvtCalc_lDvt)  "<L0_C0>"
  Bus Selector2/2 -> Right Front Conner Deviation Calculation (RFCDvtCalc)/2(RFCDvtCalc_lDvt)  "<R0_C0>"
  [LLClb_bsLLSMConClb] -> Bus Selector3/1
  Bus Selector3/1 -> Right Front Conner Deviation Calculation (RFCDvtCalc)/1(RFCDvtCalc_lDvtComp_C), Left Front Conner Deviation Calculation (LFCDvtCalc)/3(LFCDvtCalc_lDvtComp_C)  "<LL_DvtComp_C>"
  Left Front Conner Deviation Calculation (LFCDvtCalc)/1(DvtCalc_lLftDvt) -> Lane Information Selection (LaneInfoSel)1/2(LaneInfoSel_facmLftLane), Bus Creator1/7  "ILftDvt"
  Right Front Conner Deviation Calculation (RFCDvtCalc)/1(DvtCalc_lRgtDvt) -> Lane Information Selection (LaneInfoSel)1/3(LaneInfoSel_facmRgtLane), Bus Creator1/8  "IRgtDvt"
  Lane Information Selection (LaneInfoSel)1/1(LaneInfoSel_facmActvLane) -> Bus Creator1/6  "lDvt"

== system LKAS/LKAS/LL/LLOn/LKA Input Processing (LKAInP)/Predicted Heading Angle Calculation (PrHdAg) ==
  PrHdAg_bsTTLCInfo : Inport
  PrdcHdAg_stLKAActvFlg : Inport  Port=2
  PrHdAg_bsInInfoSyn : Inport  Port=3
  PrHdAg_bsLKAClb : Inport  Port=4
  Add : Sum  OutDataTypeStr=single
  Add1 : Sum  OutDataTypeStr=single
  Bus Creator : BusCreator  Inputs=10
  Bus Selector : BusSelector  OutputSignals=bsLaneInfo.bsL0Info,bsVehMovInfo.ESC_VehSpd,bsLaneInfo.bsR0Info,bsSWAInfo.SW_Angle
  Bus Selector1 : BusSelector  OutputSignals=LL_HdAgPrvwT_C
  Bus Selector2 : BusSelector  OutputSignals=LFTTTLC,RGTTTLC
  Heading Angle (HdAg) : Subsystem
  Lane Information Selection (LaneInfoSel) : Subsystem
  Lane Information Selection (LaneInfoSel)1 : Subsystem
  Min : MinMax  Inputs=2
  Perdicted Heading Angle Compensation (PrdcHdAgComp) : Subsystem
  Perdicted Heading Angle from Right Lane Line (PrdcHdAgRgt) : Subsystem
  Perdicted Heading Angle from Right Lane Line (PrdcHdAgRgt)1 : Subsystem
  Predicted Heading Angle from Left Lane Line (PrdcHdAgtLft) : Subsystem
  Predicted Heading Angle from Left Lane Line (PrdcHdAgtLft)1 : Subsystem
  Saturation : Saturate  UpperLimit=2  LowerLimit=0.5
  Z Calculation (ZCalc) : Subsystem
  Z Calculation (ZCalc)1 : Subsystem
  PrHdAg_bsPrHdAgInfo : Outport
  wires:
  Min/1 -> Saturation/1
  Bus Selector/4 -> Perdicted Heading Angle Compensation (PrdcHdAgComp)/2(PrdcHdAgComp_phiSWA)  "<SW_Angle>"
  Bus Selector/3 -> Perdicted Heading Angle from Right Lane Line (PrdcHdAgRgt)1/2(PrdcHdAgRgt_bsR0Info), Perdicted Heading Angle from Right Lane Line (PrdcHdAgRgt)/2(PrdcHdAgRgt_bsR0Info)  "<bsR0Info>"
  Bus Selector/2 -> Z Calculation (ZCalc)1/1(ZCalc_vVehSpd), Perdicted Heading Angle Compensation (PrdcHdAgComp)/1(PrdcHdAgComp_vVehSpd), Z Calculation (ZCalc)/1(ZCalc_vVehSpd)  "<ESC_VehSpd>"
  PrHdAg_bsInInfoSyn/1 -> Heading Angle (HdAg)/1(HdAg_bsLaneInfo), Bus Selector/1
  Bus Creator/1 -> PrHdAg_bsPrHdAgInfo/1
  Perdicted Heading Angle from Right Lane Line (PrdcHdAgRgt)/1(PrdcHdAgRgt_phiPrdcHdAgRgt) -> Bus Creator/4, Lane Information Selection (LaneInfoSel)1/3(LaneInfoSel_facmRgtLane), Add1/1  "phiPrvwTTLCHdAgRgt"
  Predicted Heading Angle from Left Lane Line (PrdcHdAgtLft)/1(PrdcHdAgtLft_phiPrdcHdAgLft) -> Lane Information Selection (LaneInfoSel)1/2(LaneInfoSel_facmLftLane), Bus Creator/3, Add/1  "phiPrvwTTLCHdAgLft"
  Perdicted Heading Angle Compensation (PrdcHdAgComp)/1(PrdcHdAgComp_phiPrdcHdAgComp) -> Add/2, Bus Creator/5, Add1/2  "phiPrdcHdAgComp"
  Add/1 -> Lane Information Selection (LaneInfoSel)/2(LaneInfoSel_facmLftLane)  "phiPrdcHdAgLft"
  Add1/1 -> Lane Information Selection (LaneInfoSel)/3(LaneInfoSel_facmRgtLane)  "phiPrdcHdAgRgt"
  PrdcHdAg_stLKAActvFlg/1 -> Lane Information Selection (LaneInfoSel)1/1(LaneInfoSel_stLKAActvFlg), Lane Information Selection (LaneInfoSel)/1(LaneInfoSel_stLKAActvFlg)
  Lane Information Selection (LaneInfoSel)/1(LaneInfoSel_facmActvLane) -> Bus Creator/1  "phiPrdcTTLCHdAg"
  Z Calculation (ZCalc)/1(ZCalc_lPrvwDstZ) -> Perdicted Heading Angle from Right Lane Line (PrdcHdAgRgt)/1(PrdcHdAgRgt_lPrvwDstZ), Predicted Heading Angle from Left Lane Line (PrdcHdAgtLft)/2(PrdcHdAgtLft_lPrvwDstZ)
  Bus Selector/1 -> Predicted Heading Angle from Left Lane Line (PrdcHdAgtLft)1/1(PrdcHdAgtLft_bsL0Info), Predicted Heading Angle from Left Lane Line (PrdcHdAgtLft)/1(PrdcHdAgtLft_bsL0Info)  "<bsL0Info>"
  Lane Information Selection (LaneInfoSel)1/1(LaneInfoSel_facmActvLane) -> Bus Creator/2  "phiPrvwTTLCHdAg"
  PrHdAg_bsTTLCInfo/1 -> Bus Selector2/1
  Bus Selector2/1 -> Min/1  "<LFTTTLC>"
  Bus Selector2/2 -> Min/2  "<RGTTTLC>"
  Saturation/1 -> Z Calculation (ZCalc)/2(ZCalc_tiHdAgPrvwT_C), Perdicted Heading Angle Compensation (PrdcHdAgComp)/3(PrdcHdAgComp_tiHdAgPrvwT_C)
  Heading Angle (HdAg)/1(HdAg_phiHdAg) -> Bus Creator/6  "phiHdAg"
  Heading Angle (HdAg)/2(HdAg_phiHdAgLft) -> Bus Creator/7  "phiHdAgLft"
  Heading Angle (HdAg)/3(HdAg_phiHdAgRgt) -> Bus Creator/8  "phiHdAgRgt"
  PrHdAg_bsLKAClb/1 -> Bus Selector1/1
  Bus Selector1/1 -> Z Calculation (ZCalc)1/2(ZCalc_tiHdAgPrvwT_C)  "<LL_HdAgPrvwT_C>"
  Z Calculation (ZCalc)1/1(ZCalc_lPrvwDstZ) -> Perdicted Heading Angle from Right Lane Line (PrdcHdAgRgt)1/1(PrdcHdAgRgt_lPrvwDstZ), Predicted Heading Angle from Left Lane Line (PrdcHdAgtLft)1/2(PrdcHdAgtLft_lPrvwDstZ)
  Predicted Heading Angle from Left Lane Line (PrdcHdAgtLft)1/1(PrdcHdAgtLft_phiPrdcHdAgLft) -> Bus Creator/9  "phiPrvwHdAgLft"
  Perdicted Heading Angle from Right Lane Line (PrdcHdAgRgt)1/1(PrdcHdAgRgt_phiPrdcHdAgRgt) -> Bus Creator/10  "phiPrvwHdAgRgt"

== system LKAS/LKAS/LL/LLOn/LKA Input Processing (LKAInP)/Previewed Curvature (PrCrvt) ==
  PrvwCrvt_stLKAActvFlg : Inport
  PrvwCrvt_bsInInfoSyn : Inport  Port=2
  PrvwCrvt_tiCrvtPrvwT_C : Inport  Port=3
  Bus Creator : BusCreator  Inputs=3
  Bus Selector : BusSelector  OutputSignals=LL_CrvtPrvwT_C
  Bus Selector2 : BusSelector  OutputSignals=bsLaneInfo.bsL0Info,bsVehMovInfo.ESC_VehSpd,bsLaneInfo.bsR0Info
  Curvature Ahead of Left Lane Line (CrvtAhdLft) : Subsystem
  Curvature Ahead of Left Lane Line (CrvtAhdLft)1 : Subsystem
  Lane Information Selection (LaneInfoSel) : Subsystem
  Z Calculation (ZCalc) : Subsystem
  PrvwCrvt_bsPrvwCrvtInfo : Outport
  wires:
  PrvwCrvt_bsInInfoSyn/1 -> Bus Selector2/1
  Z Calculation (ZCalc)/1(ZCalc_lPrvwDstZ) -> Curvature Ahead of Left Lane Line (CrvtAhdLft)1/1(CrvtAhdRgt_lPrvwDstZ), Curvature Ahead of Left Lane Line (CrvtAhdLft)/2(CrvtAhdLft_lPrvwDstZ)
  Bus Selector2/1 -> Curvature Ahead of Left Lane Line (CrvtAhdLft)/1(CrvtAhdLft_bsL0Info)  "<bsL0Info>"
  Bus Selector2/3 -> Curvature Ahead of Left Lane Line (CrvtAhdLft)1/2(CrvtAhdRgt_bsR0Info)  "<bsR0Info>"
  Bus Selector2/2 -> Z Calculation (ZCalc)/1(ZCalc_vVehSpd)  "<ESC_VehSpd>"
  PrvwCrvt_tiCrvtPrvwT_C/1 -> Bus Selector/1
  Bus Selector/1 -> Z Calculation (ZCalc)/2(ZCalc_tiCrvtPrvwT_C)  "<LL_CrvtPrvwT_C>"
  PrvwCrvt_stLKAActvFlg/1 -> Lane Information Selection (LaneInfoSel)/1(LaneInfoSel_stLKAActvFlg)
  Curvature Ahead of Left Lane Line (CrvtAhdLft)/1(CrvtAhdLft_crCrvtAhdLft) -> Bus Creator/2, Lane Information Selection (LaneInfoSel)/2(LaneInfoSel_facmLftLane)  "crPrvwCrvtLft"
  Curvature Ahead of Left Lane Line (CrvtAhdLft)1/1(CrvtAhdRgt_crCrvtAhdRgt) -> Lane Information Selection (LaneInfoSel)/3(LaneInfoSel_facmRgtLane), Bus Creator/3  "crPrvwCrvtRgt"
  Lane Information Selection (LaneInfoSel)/1(LaneInfoSel_facmActvLane) -> Bus Creator/1  "crPrvwCrvt"
  Bus Creator/1 -> PrvwCrvt_bsPrvwCrvtInfo/1

== system LKAS/LKAS/LL/LLOn/LKA Input Processing (LKAInP)/Steering Wheel Position Calculation (SWAPosCal) ==
  SWAPosCal_bsInInfoSyn : Inport
  Bus Selector : BusSelector  OutputSignals=bsLaneInfo.bsL0Info,bsLaneInfo.bsR0Info,bsVehMovInfo.ESC_VehSpd,bsSWAInfo.SW_Angle
  Bus Selector2 : BusSelector  OutputSignals=LKA_SampleTime
  Subsystem : Subsystem
  Subsystem1 : Subsystem
  SWAPosCal : Outport
  wires:
  SWAPosCal_bsInInfoSyn/1 -> Bus Selector/1
  Bus Selector/1 -> Subsystem1/1(L0)  "<bsL0Info>"
  Bus Selector/2 -> Subsystem1/2(R0)  "<bsR0Info>"
  Subsystem1/1(Flg) -> Subsystem/Enable  "SWAPosEna"
  Bus Selector/3 -> Subsystem1/3(VehSpd)  "<ESC_VehSpd>"
  Bus Selector/4 -> Subsystem/1(SWAIn), Subsystem1/4(SWA)  "<SW_Angle>"
  Subsystem/1(SWAPos) -> SWAPosCal/1
  [LLClb_bsConstantClb] -> Bus Selector2/1
  Bus Selector2/1 -> Subsystem/2(<LKA_SampleTime>)  "<LKA_SampleTime>"

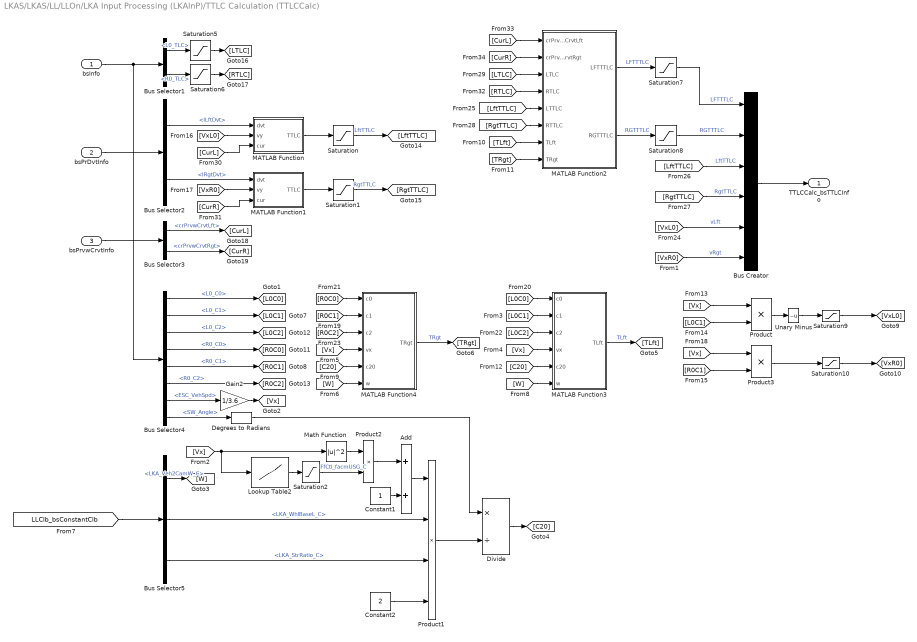
== system LKAS/LKAS/LL/LLOn/LKA Input Processing (LKAInP)/TTLC Calculation (TTLCCalc) ==
  bsInfo : Inport
  bsPrDvtInfo : Inport  Port=2
  bsPrvwCrvtInfo : Inport  Port=3
  Add : Sum  OutDataTypeStr=single
  Bus Creator : BusCreator  Inputs=6
  Bus Selector1 : BusSelector  OutputSignals=bsLaneInfo.bsL0Info.L0_TLC,bsLaneInfo.bsR0Info.R0_TLC
  Bus Selector2 : BusSelector  OutputSignals=ILftDvt,IRgtDvt
  Bus Selector3 : BusSelector  OutputSignals=crPrvwCrvtLft,crPrvwCrvtRgt
  Bus Selector4 : BusSelector  OutputSignals=bsLaneInfo.bsL0Info.L0_C0,bsLaneInfo.bsL0Info.L0_C1,bsLaneInfo.bsL0Info.L0_C2,bsLaneInfo.bsR0Info.R0_C0,bsLaneInfo.bsR0Info.R0_C1,bsLaneInfo.bsR0Info.R0_C2,bsVehMovInfo.ESC_VehSpd,bsSWAInfo.SW_Angle
  Bus Selector5 : BusSelector  OutputSignals=LKA_Veh2CamW_C,LKA_WhlBaseL_C,LKA_StrRatio_C
  Constant1 : Constant  OutDataTypeStr=single
  Constant2 : Constant  Value=2  OutDataTypeStr=single
  Degrees to Radians : simulink_extras/Transformations/Degrees to Radians
  Divide : Product  Inputs=*/
  Gain2 : Gain  Gain=1/3.6
  Lookup Table2 : Lookup_n-D  NumberOfTableDimensions=1  BreakpointsForDimension1=[11.7,18.83,26.98,31.98,51.04,79,86.08,90.59]  BeginIndexSearchUsingPreviousIndexResult=on  Table=[0.012141,0.005179,0.00298,0.002547,0.001715,0.001283,0.001021,0.000982]  DiagnosticForOutOfRangeInput=Warning  RemoveProtectionInput=on  InternalRulePriority=Speed  OutDataTypeStr=single  RndMeth=Simplest  InputSameDT=on
  MATLAB Function : MATLAB Function  TreatAsAtomicUnit=on
  MATLAB Function1 : MATLAB Function  TreatAsAtomicUnit=on
  MATLAB Function2 : MATLAB Function  TreatAsAtomicUnit=on
  MATLAB Function3 : MATLAB Function  TreatAsAtomicUnit=on
  MATLAB Function4 : MATLAB Function  TreatAsAtomicUnit=on
  Math Function : Math  Operator=magnitude^2  OutDataTypeStr=single  SaturateOnIntegerOverflow=on
  Product : Product
  Product1 : Product  Inputs=4  OutDataTypeStr=single
  Product2 : Product  OutDataTypeStr=single
  Product3 : Product
  Saturation : Saturate  UpperLimit=2  LowerLimit=0.6  OutDataTypeStr=single
  Saturation1 : Saturate  UpperLimit=2  LowerLimit=0.6  OutDataTypeStr=single
  Saturation10 : Saturate  UpperLimit=1  LowerLimit=-1
  Saturation2 : Saturate  UpperLimit=0.01  LowerLimit=0
  Saturation5 : Saturate  UpperLimit=2  LowerLimit=0.6
  Saturation6 : Saturate  UpperLimit=2  LowerLimit=0.6
  Saturation7 : Saturate  UpperLimit=2  LowerLimit=0.8
  Saturation8 : Saturate  UpperLimit=2  LowerLimit=0.8
  Saturation9 : Saturate  UpperLimit=1  LowerLimit=-1
  Unary Minus : UnaryMinus
  TTLCCalc_bsTTLCInfo : Outport
  wires:
  Divide/1 -> [C20]
  Bus Selector5/1 -> [W]  "<LKA_Veh2CamW_C>"
  [Vx] -> Math Function/1, Lookup Table2/1
  Gain2/1 -> [Vx]
  Degrees to Radians/1 -> Divide/1
  Bus Selector4/8 -> Degrees to Radians/1  "<SW_Angle>"
  Product1/1 -> Divide/2
  Bus Selector5/3 -> Product1/3  "<LKA_StrRatio_C>"
  Bus Selector5/2 -> Product1/2  "<LKA_WhlBaseL_C>"
  Add/1 -> Product1/1
  Bus Selector4/7 -> Gain2/1  "<ESC_VehSpd>"
  Saturation2/1 -> Product2/2  "FfCtl_facmUSG_C"
  Constant1/1 -> Add/2
  Lookup Table2/1 -> Saturation2/1
  Math Function/1 -> Product2/1
  Product2/1 -> Add/1
  [LLClb_bsConstantClb] -> Bus Selector5/1
  bsInfo/1 -> Bus Selector1/1, Bus Selector4/1
  bsPrDvtInfo/1 -> Bus Selector2/1
  bsPrvwCrvtInfo/1 -> Bus Selector3/1
  Saturation6/1 -> [RTLC]
  Saturation5/1 -> [LTLC]
  Bus Selector1/1 -> Saturation5/1  "<L0_TLC>"
  Bus Selector1/2 -> Saturation6/1  "<R0_TLC>"
  Bus Selector2/2 -> MATLAB Function1/1(dvt)  "<IRgtDvt>"
  [VxL0] -> MATLAB Function/2(vy)
  [VxR0] -> MATLAB Function1/2(vy)
  MATLAB Function1/1(TTLC) -> Saturation1/1
  MATLAB Function/1(TTLC) -> Saturation/1
  Saturation/1 -> [LftTTLC]  "LftTTLC"
  Saturation1/1 -> [RgtTTLC]  "RgtTTLC"
  Bus Selector2/1 -> MATLAB Function/1(dvt)  "<ILftDvt>"
  [CurR] -> MATLAB Function1/3(cur)
  [CurL] -> MATLAB Function/3(cur)
  Bus Selector3/1 -> [CurL]  "<crPrvwCrvtLft>"
  Bus Selector3/2 -> [CurR]  "<crPrvwCrvtRgt>"
  Bus Selector4/5 -> [R0C1]  "<R0_C1>"
  Bus Selector4/4 -> [R0C0]  "<R0_C0>"
  Bus Selector4/6 -> [R0C2]  "<R0_C2>"
  Bus Selector4/2 -> [L0C1]  "<L0_C1>"
  Bus Selector4/1 -> [L0C0]  "<L0_C0>"
  Bus Selector4/3 -> [L0C2]  "<L0_C2>"
  [C20] -> MATLAB Function3/5(c20)
  MATLAB Function4/1(TRgt) -> [TRgt]  "TRgt"
  [R0C2] -> MATLAB Function4/3(c2)
  [Vx] -> MATLAB Function3/4(vx)
  [C20] -> MATLAB Function4/5(c20)
  [W] -> MATLAB Function4/6(w)
  [R0C0] -> MATLAB Function4/1(c0)
  MATLAB Function3/1(TLft) -> [TLft]  "TLft"
  [L0C1] -> MATLAB Function3/2(c1)
  [W] -> MATLAB Function3/6(w)
  [R0C1] -> MATLAB Function4/2(c1)
  [Vx] -> MATLAB Function4/4(vx)
  [L0C2] -> MATLAB Function3/3(c2)
  [L0C0] -> MATLAB Function3/1(c0)
  Product3/1 -> Saturation10/1
  [Vx] -> Product3/1
  [L0C1] -> Product/2
  [Vx] -> Product/1
  Saturation9/1 -> [VxL0]
  Product/1 -> Unary Minus/1
  [R0C1] -> Product3/2
  Unary Minus/1 -> Saturation9/1
  Saturation10/1 -> [VxR0]
  [VxR0] -> Bus Creator/6  "vRgt"
  [VxL0] -> Bus Creator/5  "vLft"
  Bus Creator/1 -> TTLCCalc_bsTTLCInfo/1
  [TLft] -> MATLAB Function2/7(TLft)
  [LftTTLC] -> MATLAB Function2/5(LTTLC)
  [TRgt] -> MATLAB Function2/8(TRgt)
  [LftTTLC] -> Bus Creator/3  "LftTTLC"
  Saturation7/1 -> Bus Creator/1  "LFTTTLC"
  [CurL] -> MATLAB Function2/1(crPrvwCrvtLft)
  MATLAB Function2/1(LFTTTLC) -> Saturation7/1  "LFTTTLC"
  [RTLC] -> MATLAB Function2/4(RTLC)
  [RgtTTLC] -> Bus Creator/4  "RgtTTLC"
  [RgtTTLC] -> MATLAB Function2/6(RTTLC)
  [LTLC] -> MATLAB Function2/3(LTLC)
  MATLAB Function2/2(RGTTTLC) -> Saturation8/1  "RGTTTLC"
  Saturation8/1 -> Bus Creator/2  "RGTTTLC"
  [CurR] -> MATLAB Function2/2(crPrvwCrvtRgt)
  Constant2/1 -> Product1/4

== system LKAS/LKAS/LL/LLOn/LKA Input Processing (LKAInP)/Under The Limit (UndrLim) ==
  UndrLim_bsInInfoSyn : Inport
  UndrLim_bsUndrLimClb : Inport  Port=2
  Bus Selector : BusSelector  OutputSignals=LL_LAccMax_C,LL_LAccRMax_C
  Bus Selector1 : BusSelector  OutputSignals=bsVehMovInfo.ESC_VehSpd
  Bus Selector2 : BusSelector  OutputSignals=LKA_StrRatio_C,LKA_WhlBaseL_C
  Saturation : Saturate  UpperLimit=150  LowerLimit=0.001
  Steering Wheel Angel Max (SWAMax) : Subsystem
  Steering Wheel Angel Rate Max (SWARMax) : Subsystem
  UndrLim_phiSWAMax : Outport
  UndrLim_dphiSWARMax : Outport  Port=2
  wires:
  Saturation/1 -> Steering Wheel Angel Rate Max (SWARMax)/1(SWARateMax_vVehSpd), Steering Wheel Angel Max (SWAMax)/1(SWAMax_vVehSpd)
  Steering Wheel Angel Rate Max (SWARMax)/1(SWARMax_dphiSWARMax) -> UndrLim_dphiSWARMax/1
  Steering Wheel Angel Max (SWAMax)/1(SWAMax_phiSWAMax) -> UndrLim_phiSWAMax/1
  UndrLim_bsUndrLimClb/1 -> Bus Selector/1
  Bus Selector/1 -> Steering Wheel Angel Max (SWAMax)/2(SWAMax_aLAcc_C)  "<LL_LAccMax_C>"
  Bus Selector/2 -> Steering Wheel Angel Rate Max (SWARMax)/2(SWARateMax_aLAccR_C)  "<LL_LAccRMax_C>"
  UndrLim_bsInInfoSyn/1 -> Bus Selector1/1
  Bus Selector1/1 -> Saturation/1  "<ESC_VehSpd>"
  Bus Selector2/1 -> Steering Wheel Angel Max (SWAMax)/3(LKA_StrRatio_C), Steering Wheel Angel Rate Max (SWARMax)/3(LKA_StrRatio_C)  "<LKA_StrRatio_C>"
  Bus Selector2/2 -> Steering Wheel Angel Max (SWAMax)/4(LKA_WhlBaseL_C), Steering Wheel Angel Rate Max (SWARMax)/4(LKA_WhlBaseL_C)  "<LKA_WhlBaseL_C>"
  [LLClb_bsConstantClb] -> Bus Selector2/1
